simulink model "Subsystem"  (R2019b)
settings: Solver=FixedStepAuto  StartTime=0.0  StopTime=testtime  RelTol=1e-3
InitFcn:
  | OHC_Lowpass_Test_Parameters
StopFcn:
  | Verify_OHC_Lowpass_Filter
undefined symbols (not defined in the file or in its folder): OHCLPcoeffs
settings Model: Creator=mblun
settings DataIOCC: SaveOutput=off  SaveTime=off
settings OptimizationCC: BlockReduction=off  ConditionallyExecuteInputs=off  DefaultParameterBehavior=Inlined
settings DebuggingCC: AlgebraicLoopMsg=error
settings HardwareCC: ProdBitPerPointer=32  ProdBitPerSizeT=32  ProdBitPerPtrDiffT=32  ProdLargestAtomicFloat=None  ProdIntDivRoundTo=Undefined  ProdEndianess=Unspecified  ProdWordSize=32  ProdHWDeviceType=ASIC/FPGA->ASIC/FPGA  TargetBitPerPointer=64  TargetBitPerSizeT=64  TargetBitPerPtrDiffT=64  TargetLongLongMode=on  TargetIntDivRoundTo=Zero  TargetEndianess=LittleEndian  TargetWordSize=64  TargetHWDeviceType=Custom Processor->MATLAB Host Computer  ProdEqTarget=off
settings SFSimCC: CustomCodeUndefinedFunction=UseInterfaceOnly

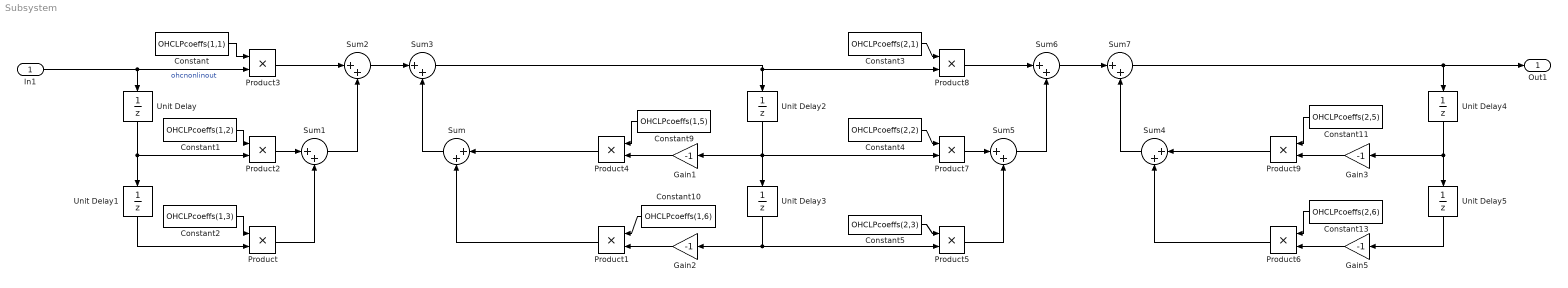
== system Subsystem ==
  In1 : Inport  OutDataTypeStr=single  PortDimensions=[1 1]  SampleTime=[2.0833333333333333e-05,0]
  Constant : Constant  Value=OHCLPcoeffs(1,1)  OutDataTypeStr=single  SampleTime=-1
  Constant1 : Constant  Value=OHCLPcoeffs(1,2)  OutDataTypeStr=single  SampleTime=-1
  Constant10 : Constant  Value=OHCLPcoeffs(1,6)  OutDataTypeStr=single  SampleTime=-1
  Constant11 : Constant  Value=OHCLPcoeffs(2,5)  OutDataTypeStr=single  SampleTime=-1
  Constant13 : Constant  Value=OHCLPcoeffs(2,6)  OutDataTypeStr=single  SampleTime=-1
  Constant2 : Constant  Value=OHCLPcoeffs(1,3)  OutDataTypeStr=single  SampleTime=-1
  Constant3 : Constant  Value=OHCLPcoeffs(2,1)  OutDataTypeStr=single  SampleTime=-1
  Constant4 : Constant  Value=OHCLPcoeffs(2,2)  OutDataTypeStr=single  SampleTime=-1
  Constant5 : Constant  Value=OHCLPcoeffs(2,3)  OutDataTypeStr=single  SampleTime=-1
  Constant9 : Constant  Value=OHCLPcoeffs(1,5)  OutDataTypeStr=single  SampleTime=-1
  Gain{1..3,5} (4 alike) : Gain  Gain=-1
  Product{,1..9} (10 alike) : Product
  Sum{,1..7} (8 alike) : Sum  Inputs=|++
  Unit Delay{,1..5} (6 alike) : UnitDelay  SampleTime=-1  HasFrameUpgradeWarning=on
  Out1 : Outport  OutDataTypeStr=single  PortDimensions=1  SampleTime=[2.0833333333333333e-05,0]
  wires:
  Constant2/1 -> Product/1
  Unit Delay/1 -> Product2/2, Unit Delay1/1
  Sum1/1 -> Sum2/2
  Constant3/1 -> Product8/1
  Constant13/1 -> Product6/1
  Constant/1 -> Product3/1
  Constant1/1 -> Product2/1
  Constant9/1 -> Product4/1
  Unit Delay2/1 -> Gain1/1, Unit Delay3/1, Product7/2
  In1/1 -> Unit Delay/1, Product3/2  "ohcnonlinout"
  Sum5/1 -> Sum6/2
  Constant10/1 -> Product1/1
  Unit Delay4/1 -> Gain3/1, Unit Delay5/1
  Product7/1 -> Sum5/1
  Gain1/1 -> Product4/2
  Constant4/1 -> Product7/1
  Product3/1 -> Sum2/1
  Product2/1 -> Sum1/1
  Product5/1 -> Sum5/2
  Constant5/1 -> Product5/1
  Unit Delay3/1 -> Gain2/1, Product5/2
  Unit Delay1/1 -> Product/2
  Unit Delay5/1 -> Gain5/1
  Product8/1 -> Sum6/1
  Gain2/1 -> Product1/2
  Gain3/1 -> Product9/2
  Gain5/1 -> Product6/2
  Constant11/1 -> Product9/1
  Product/1 -> Sum1/2
  Sum2/1 -> Sum3/1
  Sum6/1 -> Sum7/1
  Product4/1 -> Sum/1
  Product1/1 -> Sum/2
  Product9/1 -> Sum4/1
  Product6/1 -> Sum4/2
  Sum/1 -> Sum3/2
  Sum3/1 -> Unit Delay2/1, Product8/2
  Sum4/1 -> Sum7/2
  Sum7/1 -> Out1/1, Unit Delay4/1
